simulink model "steam_force"  (Simulink 7.6)
settings: Solver=ode45  StartTime=0.0  StopTime=50.0  RelTol=1e-3
libraries: simulink x1
settings Model: Creator=pogilvie  LastModifiedBy=pogilvie
settings OptimizationCC: InitFltsAndDblsToZero=on
settings DebuggingCC: SaveWithParameterizedLinksMsg=none  SignalResolutionControl=TryResolveAllWithWarning  StrictBusMsg=Warning
settings GRTTargetCC: TargetFcnLib=ansi_tfl_tmw.mat

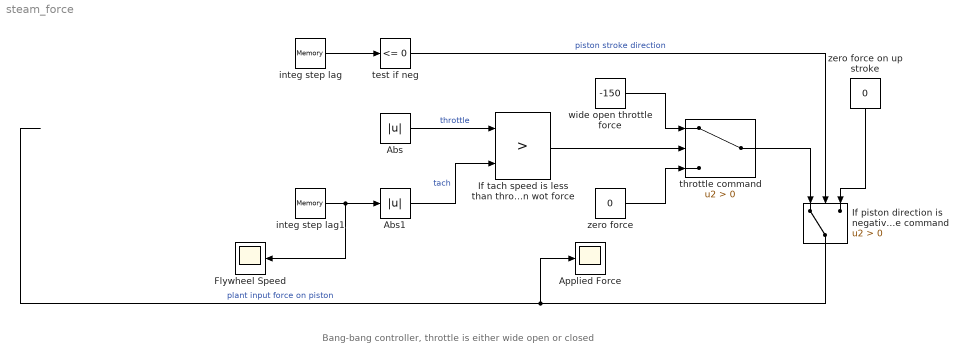
== system steam_force ==
  note: Bang-bang controller, throttle is either wide open or closed
  Abs : Abs
  Abs1 : Abs
  Applied Force : Scope
  Flywheel Speed : Scope
  If piston direction is negative (down stroke) then use throttle command : Switch  Criteria=u2 > Threshold
  If tach speed is less than throttle then turn on wot force : RelationalOperator  Operator=>  OutDataTypeStr=boolean
  integ step lag : Memory  InheritSampleTime=on
  integ step lag1 : Memory  InheritSampleTime=on
  test if neg : simulink/Logic and Bit Operations/Compare To Constant  SystemSampleTime=-1  relop=<=  const=0  LogicOutDataTypeMode=uint8  ZeroCross=off
  throttle command : Switch  Criteria=u2 > Threshold
  wide open throttle force : Constant  Value=-150
  zero force : Constant  Value=0
  zero force on up stroke : Constant  Value=0
  wires:
  zero force on up stroke/1 -> If piston direction is negative (down stroke) then use throttle command/3
  test if neg/1 -> If piston direction is negative (down stroke) then use throttle command/2  "piston stroke direction"
  throttle command/1 -> If piston direction is negative (down stroke) then use throttle command/1
  wide open throttle force/1 -> throttle command/1
  zero force/1 -> throttle command/3
  If tach speed is less than throttle then turn on wot force/1 -> throttle command/2
  ? -> integ step lag/1  "p out piston vel"
  If piston direction is negative (down stroke) then use throttle command/1 -> Applied Force/1  "plant input force on piston"
  Abs1/1 -> If tach speed is less than throttle then turn on wot force/2  "tach"
  ? -> integ step lag1/1  "p out flywheel speed"
  ? -> Abs/1  "p out desired speed"
  Abs/1 -> If tach speed is less than throttle then turn on wot force/1  "throttle"
  integ step lag/1 -> test if neg/1
  integ step lag1/1 -> Abs1/1, Flywheel Speed/1
